simulink model "rct_pendulum_pluspos"  (R2023a)
settings: Solver=FixedStepAuto  StartTime=0.0  StopTime=30  FixedStep=0.00005  MaxStep=1e-5  RelTol=1e-5  EnableMultiTasking=on
model workspace (MATLAB code in the model file):
  | mCart = 1;
  | mPend = 1;
  | g = 9.81;
  | L = 0.5;
  | theta0 = 0;
  | Kd = 10;
undefined symbols (not defined in the file): X, Y, Z
libraries: sm_lib x11, nesl_utility x5
settings Model: Creator=The MathWorks, Inc.  LastModifiedBy=kimdi
settings SolverCC: AlgebraicLoopSolver=TrustRegion  MaxZcPerStep=1
settings DataIOCC: LimitDataPoints=on  SaveFormat=Array  ReturnWorkspaceOutputs=off  OutputOption=SpecifiedOutputTimes  OutputTimes=0:1/30:12
settings OptimizationCC: ReuseModelBlockBuffer=off  LifeSpan=inf
settings DebuggingCC: UnderspecifiedInitializationDetection=Classic  MergeDetectMultiDrivingBlocksExec=none  SolverPrmCheckMsg=warning  UnconnectedInputMsg=warning  UnconnectedOutputMsg=warning  UnconnectedLineMsg=warning  StateNameClashWarn=warning  SFUnexpectedBacktrackingDiag=warning  SFNoUnconditionalDefaultTransitionDiag=warning  SFExecutionAtInitializationDiag=none  ArithmeticOperatorsInVariantConditions=warning
settings HardwareCC: ProdBitPerPointer=32  ProdBitPerSizeT=32  ProdBitPerPtrDiffT=32  ProdLargestAtomicFloat=None  ProdIntDivRoundTo=Undefined  ProdEndianess=Unspecified  ProdWordSize=32  ProdHWDeviceType=32-bit Generic
settings ModelReferenceCC: EnableRefExpFcnMdlSchedulingChecks=on  PropagateSignalLabelsOutOfModel=off
settings SFSimCC: SimUseLocalCustomCode=off  CustomCodeUndefinedFunction=UseInterfaceOnly
settings RTWCC: RTWUseLocalCustomCode=off  DLArmComputeVersion=19.05
settings CodeAppCC: StateflowObjectComments=on
settings GRTTargetCC: TargetLangStandard=C89/C90 (ANSI)
settings ConfigComp: CovMetricSettings=dw  CovSaveCumulativeToWorkspaceVar=on  CovSaveSingleToWorkspaceVar=on  CovExternalEMLEnable=off  CovSFcnEnable=off
settings SimscapeCC: SimscapeNormalizeSystem=off
settings ConfigurationSet: Description=SimMechanics 2G
settings ExplorerConfigSet: InternalSimMechanicsExplorerSettings="<ExplorerConfiguration><canonicalview>default</canonicalview><TilePanel><TileInfo><Tiles Columns=\"1\" Count=\"1\" Rows=\"1\"><Column Left=\"2\" Weight=\"1\"/><Column Left=\"591\"/><Row Top=\"2\" Weight=\"1\"/><Row Top=\"389\"/><Tile Height=\"1\" Width=\"1\" X=\"0\" Y=\"0\"/></Tiles></TileInfo><SceneInfo><SceneViewer><BGColor><R>0.60000002384185791</R><G>0.60000002384185791</G><B>0.60000002384185791</B></BGColor><Camera><Position><X>0.64243946887929204</X><Y>-49.663614699976236</Y><Z>0.22319801622928798</Z></Position><Center><X>0.64243946887929204</X><Y>0</Y><Z>0.22319801622928798</Z></Center><Up><X>0</X><Y>-0</Y><Z>1</Z></Up><Left>-0.88124258449330872</Left><Right>0.88124258449330872</Right><Bottom>-0.30475961919215644</Bottom><Top>0.30475961919215644</Top></Camera></SceneViewer></SceneInfo></TilePanel></ExplorerConfiguration>"

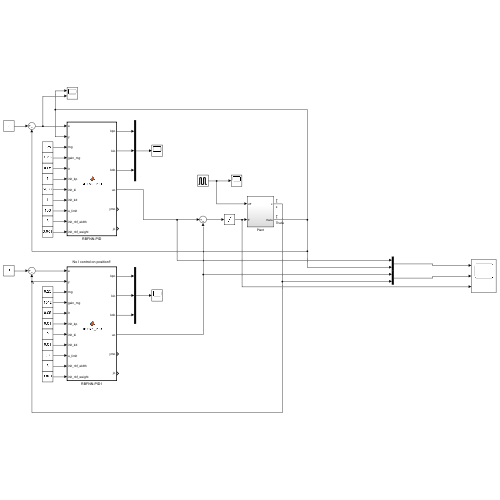
[thumbnail: Simulink's stored preview of the top-level diagram]
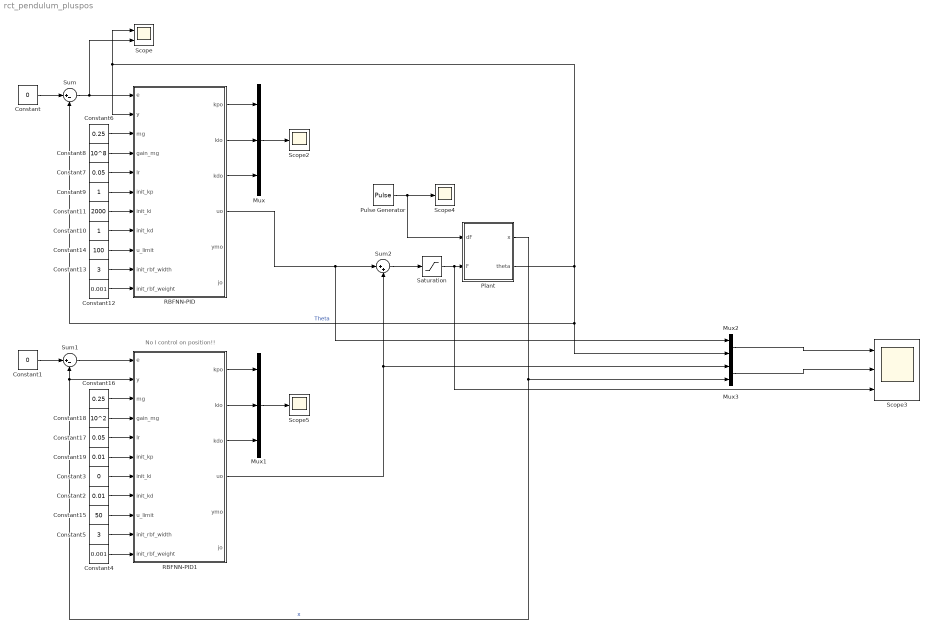
== system rct_pendulum_pluspos ==
  note: No I control on position!!
  Constant : Constant  Value=0
  Constant1 : Constant  Value=0
  Constant10 : Constant
  Constant11 : Constant  Value=2000
  Constant12 : Constant  Value=0.001
  Constant13 : Constant  Value=3
  Constant14 : Constant  Value=100
  Constant15 : Constant  Value=50
  Constant16 : Constant  Value=0.25
  Constant17 : Constant  Value=0.05
  Constant18 : Constant  Value=10^2
  Constant19 : Constant  Value=0.01
  Constant2 : Constant  Value=0.01
  Constant3 : Constant  Value=0
  Constant4 : Constant  Value=0.001
  Constant5 : Constant  Value=3
  Constant6 : Constant  Value=0.25
  Constant7 : Constant  Value=0.05
  Constant8 : Constant  Value=10^8
  Constant9 : Constant
  Mux : Mux  Inputs=3
  Mux1 : Mux  Inputs=3
  Mux2 : Mux  Inputs=2
  Mux3 : Mux  Inputs=2
  Plant : Subsystem
  Pulse Generator : DiscretePulseGenerator  PulseType=Time based  Period=10  PulseWidth=5  PhaseDelay=3
  RBFNN-PID : MATLAB Function  TreatAsAtomicUnit=on
  RBFNN-PID1 : MATLAB Function  TreatAsAtomicUnit=on
  Saturation : Saturate  UpperLimit=1000  LowerLimit=-1000
  Scope : Scope  NumInputPorts=2
  Scope2 : Scope
  Scope3 : Scope  NumInputPorts=3
  Scope4 : Scope
  Scope5 : Scope
  Sum : Sum  Inputs=|+-
  Sum1 : Sum  Inputs=|+-
  Sum2 : Sum  Inputs=|++
  wires:
  Constant/1 -> Sum/1
  Sum/1 -> RBFNN-PID/1(e), Scope/2
  Plant/2(theta) -> RBFNN-PID/2(y), Scope/1, Sum/2, Mux2/2  "Theta"
  Mux/1 -> Scope2/1
  RBFNN-PID/1(kpo) -> Mux/1
  RBFNN-PID/2(kio) -> Mux/2
  RBFNN-PID/3(kdo) -> Mux/3
  Constant1/1 -> Sum1/1
  Sum1/1 -> RBFNN-PID1/1(e)
  Plant/1(x) -> RBFNN-PID1/2(y), Sum1/2, Mux3/2  "x"
  RBFNN-PID1/3(kdo) -> Mux1/3
  Mux1/1 -> Scope5/1
  RBFNN-PID1/2(kio) -> Mux1/2
  RBFNN-PID1/1(kpo) -> Mux1/1
  RBFNN-PID/4(uo) -> Sum2/1, Mux2/1
  RBFNN-PID1/4(uo) -> Mux3/1, Sum2/2
  Mux2/1 -> Scope3/1
  Mux3/1 -> Scope3/2
  Pulse Generator/1 -> Plant/1(dF), Scope4/1
  Saturation/1 -> Scope3/3, Plant/2(F)
  Sum2/1 -> Saturation/1
  Constant6/1 -> RBFNN-PID/3(mg)
  Constant8/1 -> RBFNN-PID/4(gain_mg)
  Constant7/1 -> RBFNN-PID/5(lr)
  Constant9/1 -> RBFNN-PID/6(init_kp)
  Constant10/1 -> RBFNN-PID/8(init_kd)
  Constant11/1 -> RBFNN-PID/7(init_ki)
  Constant13/1 -> RBFNN-PID/10(init_rbf_width)
  Constant14/1 -> RBFNN-PID/9(u_limit)
  Constant12/1 -> RBFNN-PID/11(init_rbf_weight)
  Constant16/1 -> RBFNN-PID1/3(mg)
  Constant3/1 -> RBFNN-PID1/7(init_ki)
  Constant15/1 -> RBFNN-PID1/9(u_limit)
  Constant5/1 -> RBFNN-PID1/10(init_rbf_width)
  Constant4/1 -> RBFNN-PID1/11(init_rbf_weight)
  Constant17/1 -> RBFNN-PID1/5(lr)
  Constant19/1 -> RBFNN-PID1/6(init_kp)
  Constant2/1 -> RBFNN-PID1/8(init_kd)
  Constant18/1 -> RBFNN-PID1/4(gain_mg)

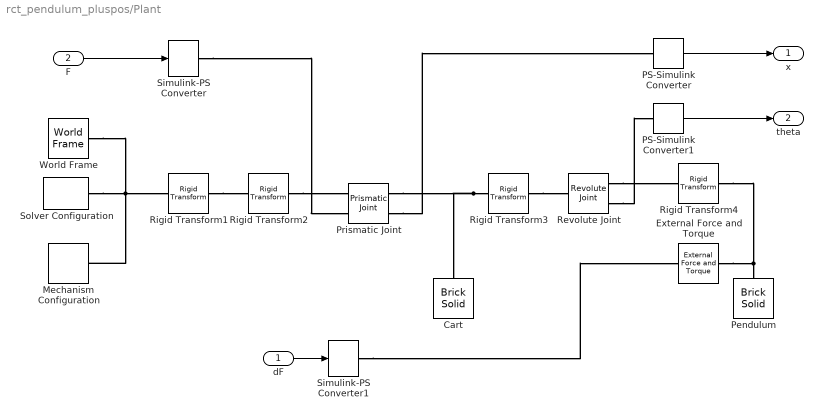
== system rct_pendulum_pluspos/Plant ==
  dF : Inport
  F : Inport  Port=2
  Cart : sm_lib/Body Elements/Brick Solid  GraphicAmbientColor=[0.15 0.15 0.15 1.0]  BasedOnType=Mass  BrickDimensions=[L/6 L/6 L/3]  BrickDimensionsUnits=m  CenterOfMass=[0 0 0]  CenterOfMassUnits=m  GraphicDiffuseColor=[0.5 0.5 0.5]  Density=1000  DensityUnits=kg/(m^3)  DoExposeReferenceFrame=on  GraphicEmissiveColor=[0.0 0.0 0.0 1.0]  ExportEntireGeometry=off  SerializedFrames=<Frames/>  MarkerShape=Sphere  MarkerSize=10  GraphicType=FromGeometry  InertiaType=PointMass  Mass=mCart  MassUnits=kg  MomentsOfInertia=[1 1 1]  MomentsOfInertiaUnits=kg*m^2  GraphicOpacity=1.0  ProductsOfInertia=[0 0 0]  ProductsOfInertiaUnits=kg*m^2  GraphicShininess=75  GraphicSpecularColor=[0.5 0.5 0.5 1.0]  GraphicVisPropType=SimpleVisualProperties
  External Force and Torque : sm_lib/Forces and Torques/External Force and Torque  ForceResolutionFrame=World  EnableForceX=on  EnableForceY=off  EnableForceZ=off  EnableForce=off  TorqueResolutionFrame=AttachedFrame  EnableTorqueX=off  EnableTorqueY=off  EnableTorqueZ=off  EnableTorque=off
  Mechanism Configuration : sm_lib/Utilities/Mechanism Configuration  UniformGravity=Constant  GravityVector=[0 0 -9.81]  GravityVectorUnits=m/s^2  LinearizationDelta=0.001  JointModeTransitionNonlinearIterations=2
  PS-Simulink Converter : nesl_utility/PS-Simulink Converter  PhysicalDomain=network_engine_domain  SubClassName=ps_output  LeftPortType=input  RightPortType=output  PseudoPeriodic=off  Frequencies=[]  VectorFormat=1-D array  Unit=1  AffineConversion=off
  PS-Simulink Converter1 : nesl_utility/PS-Simulink Converter  PhysicalDomain=network_engine_domain  SubClassName=ps_output  LeftPortType=input  RightPortType=output  PseudoPeriodic=off  Frequencies=[]  VectorFormat=1-D array  Unit=1  AffineConversion=off
  Pendulum : sm_lib/Body Elements/Brick Solid  GraphicAmbientColor=[0.15 0.15 0.15 1.0]  BasedOnType=Mass  BrickDimensions=[L L/12 L/12]  BrickDimensionsUnits=m  CenterOfMass=[0 0 0]  CenterOfMassUnits=m  GraphicDiffuseColor=[0.8 0.0 0.2]  Density=1000  DensityUnits=kg/(m^3)  DoExposeReferenceFrame=on  GraphicEmissiveColor=[0.0 0.0 0.0 1.0]  ExportEntireGeometry=off  SerializedFrames=<Frames/>  MarkerShape=Sphere  MarkerSize=10  GraphicType=FromGeometry  InertiaType=PointMass  Mass=mPend  MassUnits=kg  MomentsOfInertia=[1 1 1]  MomentsOfInertiaUnits=kg*m^2  GraphicOpacity=1.0  ProductsOfInertia=[0 0 0]  ProductsOfInertiaUnits=kg*m^2  GraphicShininess=75  GraphicSpecularColor=[0.5 0.5 0.5 1.0]  GraphicVisPropType=SimpleVisualProperties
  Prismatic Joint : sm_lib/Joints/Prismatic Joint  JointMode=Normal  SenseConstraintForce=off  SenseConstraintForceX=off  SenseConstraintForceY=off  SenseConstraintForceZ=off  SenseConstraintTorque=off  SenseConstraintTorqueX=off  SenseConstraintTorqueY=off  SenseConstraintTorqueZ=off  SenseTotalForce=off  SenseTotalForceX=off  SenseTotalForceY=off  SenseTotalForceZ=off  SenseTotalTorque=off  SenseTotalTorqueX=off  SenseTotalTorqueY=off  SenseTotalTorqueZ=off  CompositeWrenchDir=FollowerOnBase  CompositeWrenchFrame=BaseFrame  EquilibriumPosition=0  EquilibriumPositionUnits=m  SpringStiffness=0  SpringStiffnessUnits=N/m  DampingCoefficient=Kd  DampingCoefficientUnits=N/(m/s)  TorqueActuationMode=InputTorque  MotionActuationMode=ComputedMotion  SensePosition=on  SenseVelocity=off  SenseAcceleration=off  SenseTorqueForce=off  SenseLowerLimitTorqueForce=off  SenseUpperLimitTorqueForce=off  LowerLimitSpecify=off  LowerLimitBound=-1  LowerLimitBoundUnits=m  LowerLimitStiffness=1e6  LowerLimitStiffnessUnits=N/m  LowerLimitDamping=1e3  LowerLimitDampingUnits=N/(m/s)  LowerLimitTransitionRegionWidth=1e-4  LowerLimitTransitionRegionWidthUnits=m  UpperLimitSpecify=off  UpperLimitBound=1  UpperLimitBoundUnits=m  UpperLimitStiffness=1e6  UpperLimitStiffnessUnits=N/m  UpperLimitDamping=1e3  UpperLimitDampingUnits=N/(m/s)  UpperLimitTransitionRegionWidth=1e-4  UpperLimitTransitionRegionWidthUnits=m  PositionTargetSpecify=off  PositionTargetPriority=High  PositionTargetValue=0  PositionTargetValueUnits=m  VelocityTargetSpecify=off  VelocityTargetPriority=High  VelocityTargetValue=0  VelocityTargetValueUnits=m/s
  Revolute Joint : sm_lib/Joints/Revolute Joint  JointMode=Normal  SenseConstraintForce=off  SenseConstraintForceX=off  SenseConstraintForceY=off  SenseConstraintForceZ=off  SenseConstraintTorque=off  SenseConstraintTorqueX=off  SenseConstraintTorqueY=off  SenseConstraintTorqueZ=off  SenseTotalForce=off  SenseTotalForceX=off  SenseTotalForceY=off  SenseTotalForceZ=off  SenseTotalTorque=off  SenseTotalTorqueX=off  SenseTotalTorqueY=off  SenseTotalTorqueZ=off  CompositeWrenchDir=FollowerOnBase  CompositeWrenchFrame=BaseFrame  EquilibriumPosition=0  EquilibriumPositionUnits=deg  SpringStiffness=0  SpringStiffnessUnits=N*m/deg  DampingCoefficient=0  DampingCoefficientUnits=N*m/(rad/s)  TorqueActuationMode=NoTorque  MotionActuationMode=ComputedMotion  SensePosition=on  SenseVelocity=off  SenseAcceleration=off  SenseTorqueForce=off  SenseLowerLimitTorqueForce=off  SenseUpperLimitTorqueForce=off  LowerLimitSpecify=off  LowerLimitBound=-90  LowerLimitBoundUnits=deg  LowerLimitStiffness=1e4  LowerLimitStiffnessUnits=N*m/deg  LowerLimitDamping=10  LowerLimitDampingUnits=N*m/(deg/s)  LowerLimitTransitionRegionWidth=0.1  LowerLimitTransitionRegionWidthUnits=deg  UpperLimitSpecify=off  UpperLimitBound=90  UpperLimitBoundUnits=deg  UpperLimitStiffness=1e4  UpperLimitStiffnessUnits=N*m/deg  UpperLimitDamping=10  UpperLimitDampingUnits=N*m/(deg/s)  UpperLimitTransitionRegionWidth=0.1  UpperLimitTransitionRegionWidthUnits=deg  PositionTargetSpecify=on  PositionTargetPriority=High  PositionTargetValue=theta0  PositionTargetValueUnits=deg  VelocityTargetSpecify=off  VelocityTargetPriority=High  VelocityTargetValue=0  VelocityTargetValueUnits=deg/s
  Rigid Transform1 : sm_lib/Frames and Transforms/Rigid Transform  TranslationMethod=None  TranslationStandardOffset=0  TranslationStandardOffsetUnits=m  TranslationStandardAxis=+Z  TranslationCartesianOffset=[0 0 0]  TranslationCartesianOffsetUnits=m  TranslationROffset=0  TranslationROffsetUnits=m  TranslationZOffset=0  TranslationZOffsetUnits=m  TranslationThetaOffset=0  TranslationThetaOffsetUnits=deg  RotationMethod=StandardAxis  RotationAngleUnits=deg  RotationStandardAxis=+Y  RotationAngle=90  RotationArbitraryAxis=[0 0 1]  FollAlignAxisA=+X  BaseAlignAxisA=+Y  FollAlignAxisB=+Y  BaseAlignAxisB=+Z  RotationSequenceAxes=FollowerAxes  RotationSequence=XYX  RotationSequenceAngles=[0 0 0]  RotationSequenceAnglesUnits=deg  RotationMatrix=[1 0 0; 0 1 0; 0 0 1]  Quaternion=[1 0 0 0]
  Rigid Transform2 : sm_lib/Frames and Transforms/Rigid Transform  TranslationMethod=None  TranslationStandardOffset=0  TranslationStandardOffsetUnits=m  TranslationStandardAxis=+Z  TranslationCartesianOffset=[0 0 0]  TranslationCartesianOffsetUnits=m  TranslationROffset=0  TranslationROffsetUnits=m  TranslationZOffset=0  TranslationZOffsetUnits=m  TranslationThetaOffset=0  TranslationThetaOffsetUnits=deg  RotationMethod=StandardAxis  RotationAngleUnits=deg  RotationStandardAxis=+Z  RotationAngle=180  RotationArbitraryAxis=[0 0 1]  FollAlignAxisA=+X  BaseAlignAxisA=+Y  FollAlignAxisB=+Y  BaseAlignAxisB=+Z  RotationSequenceAxes=FollowerAxes  RotationSequence=XYX  RotationSequenceAngles=[0 0 0]  RotationSequenceAnglesUnits=deg  RotationMatrix=[1 0 0; 0 1 0; 0 0 1]  Quaternion=[1 0 0 0]
  Rigid Transform3 : sm_lib/Frames and Transforms/Rigid Transform  TranslationMethod=None  TranslationStandardOffset=0  TranslationStandardOffsetUnits=m  TranslationStandardAxis=+Z  TranslationCartesianOffset=[0 0 0]  TranslationCartesianOffsetUnits=m  TranslationROffset=0  TranslationROffsetUnits=m  TranslationZOffset=0  TranslationZOffsetUnits=m  TranslationThetaOffset=0  TranslationThetaOffsetUnits=deg  RotationMethod=StandardAxis  RotationAngleUnits=deg  RotationStandardAxis=-X  RotationAngle=90  RotationArbitraryAxis=[0 0 1]  FollAlignAxisA=+X  BaseAlignAxisA=+Y  FollAlignAxisB=+Y  BaseAlignAxisB=+Z  RotationSequenceAxes=FollowerAxes  RotationSequence=XYX  RotationSequenceAngles=[0 0 0]  RotationSequenceAnglesUnits=deg  RotationMatrix=[1 0 0; 0 1 0; 0 0 1]  Quaternion=[1 0 0 0]
  Rigid Transform4 : sm_lib/Frames and Transforms/Rigid Transform  TranslationMethod=StandardAxis  TranslationStandardOffset=L/2  TranslationStandardOffsetUnits=m  TranslationStandardAxis=+X  TranslationCartesianOffset=[0 0 0]  TranslationCartesianOffsetUnits=m  TranslationROffset=0  TranslationROffsetUnits=m  TranslationZOffset=0  TranslationZOffsetUnits=m  TranslationThetaOffset=0  TranslationThetaOffsetUnits=deg  RotationMethod=StandardAxis  RotationAngleUnits=deg  RotationStandardAxis=+X  RotationAngle=90  RotationArbitraryAxis=[0 0 1]  FollAlignAxisA=+X  BaseAlignAxisA=+Y  FollAlignAxisB=+Y  BaseAlignAxisB=+Z  RotationSequenceAxes=FollowerAxes  RotationSequence=XYX  RotationSequenceAngles=[0 0 0]  RotationSequenceAnglesUnits=deg  RotationMatrix=[1 0 0; 0 1 0; 0 0 1]  Quaternion=[1 0 0 0]
  Simulink-PS Converter : nesl_utility/Simulink-PS Converter  PhysicalDomain=network_engine_domain  SubClassName=ps_input  LeftPortType=input  RightPortType=output  PseudoPeriodic=off  Frequencies=[]  NoiseDistribution=none  NoiseParameters=[]  Unit=1  AffineConversion=off  FilteringAndDerivatives=zero  SimscapeFilterOrder=1  InputFilterTimeConstant=0.001  UdotUserProvided=1
  Simulink-PS Converter1 : nesl_utility/Simulink-PS Converter  PhysicalDomain=network_engine_domain  SubClassName=ps_input  LeftPortType=input  RightPortType=output  PseudoPeriodic=off  Frequencies=[]  NoiseDistribution=none  NoiseParameters=[]  Unit=1  AffineConversion=off  FilteringAndDerivatives=zero  SimscapeFilterOrder=1  InputFilterTimeConstant=0.001  UdotUserProvided=1
  Solver Configuration : nesl_utility/Solver Configuration  PhysicalDomain=network_engine_domain  SubClassName=solver  LeftPortType=input  RightPortType=generic  Tones=[]  Harmonics=[]  SimulateNoise=off  Profile=off  UseLocalSampling=off  EnableSwitchedLinearOptims=on  FrequencyDomain=off  UseCCode=off  RelTol=0.001  AbsTol=1e-06  MinStep=1e-09  ToWorkspace=off  RevertToSquareIcSolve=off  NumHomotopyIterations=100  PhasorMode=off  PhasorModeNumHarmonics=1  ConsistencySolver=NEWTON_FTOL  IndexReductionMethod=DerivativeReplacement  DoDC=off  ResidualTolerance=1e-09  ConsistencyTolSource=GLOBAL  ConsistencyAbsTol=0.001  ConsistencyRelTol=0.001  ConsistencyTolFactor=0.001  UseLocalSolver=off  LocalSolverChoice=NE_BACKWARD_EULER_ADVANCER  ResolveIndetEquations=on  FunctionEvalNumThread=1  LocalSolverSampleTime=0.001  DoFixedCost=off  MaxNonlinIter=3  MaxModeIter=2  ComputeImpulses=off  ImpulseIterations=2  LinearAlgebra=Sparse  LinearAlgebraNumThread=0  EquationFormulation=NE_TIME_EF  DelaysMemoryBudget=1024  AutomaticFiltering=on  FilteringTimeConstant=0.001  PartitionStorageMethod=AS_NEEDED  PartitionMemoryBudget=1024  PartitionMethod=FAST
  World Frame : sm_lib/Frames and Transforms/World Frame
  x : Outport  VectorParamsAs1DForOutWhenUnconnected=off
  theta : Outport  Port=2  VectorParamsAs1DForOutWhenUnconnected=off
  wires:
  PS-Simulink Converter1/1 -> theta/1
  PS-Simulink Converter/1 -> x/1
  F/1 -> Simulink-PS Converter/1
  dF/1 -> Simulink-PS Converter1/1
  connections:
  Rigid Transform3/LConn1 -- Cart/RConn1 -- Prismatic Joint/RConn1
  World Frame/RConn1 -- Solver Configuration/RConn1 -- Mechanism Configuration/RConn1 -- Rigid Transform1/LConn1
  Revolute Joint/RConn1 -- Rigid Transform4/LConn1
  Rigid Transform4/RConn1 -- External Force and Torque/RConn1 -- Pendulum/RConn1
  Rigid Transform3/RConn1 -- Revolute Joint/LConn1
  Revolute Joint/RConn2 -- PS-Simulink Converter1/LConn1
  Prismatic Joint/RConn2 -- PS-Simulink Converter/LConn1
  Simulink-PS Converter/RConn1 -- Prismatic Joint/LConn2
  Simulink-PS Converter1/RConn1 -- External Force and Torque/LConn1
  Rigid Transform1/RConn1 -- Rigid Transform2/LConn1
  Rigid Transform2/RConn1 -- Prismatic Joint/LConn1

== matlab function rct_pendulum_pluspos/RBFNN-PID1 ==
  settings: updateMethod=DISCRETE
  data: e input; y input; kpo output; kio output; kdo output; mg input; gain_mg input; lr input; uo output; ymo output; jo output; init_kp input; init_ki input; init_kd input; u_limit input; init_rbf_width input; init_rbf_weight input
% e is error, PID input
% y is output of plant
% mg is momentum factor of RBF NN
% lr is learning rate of RBF NN
function [kpo, kio, kdo, uo, ymo, jo]= RBFNN_PID(e, y, mg, gain_mg, lr, init_kp, init_ki, init_kd, u_limit, init_rbf_width, init_rbf_weight)
persistent flag;

% PID controller parameters
persistent ek ek1 ek2; % e(k), e(k-1), e(k-2)
persistent sumek;
persistent xc1 xc2 xc3; % xc(1), xc(2), xc(3)
persistent u du;
persistent kp ki kd;

% RBF NN parameters
n = 3; % size of input
m = 8; % size of hidden
persistent X; % input X [n x 1]
persistent Ck Ck1 Ck2; % center vector C [m x n]
persistent H; % radial vector [m x 1]
persistent Bk Bk1 Bk2; % radial width vector B [m x 1]
persistent Wk Wk1 Wk2; % weight vector W [m x 1]
persistent yk yk1; % output of plant
persistent ym; % output of RBF NN
persistent J; % jacobian information of RBF NN

% initialize inital value just first time
if isempty(flag)
    flag = 1;

    ek1 = 0;
    ek2 = 0;
    sumek = 0;
    
    u = 0;
    du = 0;

    kp = init_kp;
    ki = init_ki;
    kd = init_kd;
    X = zeros(n, 1);
    Ck = zeros(m, n);
    Ck1 = zeros(m, n);
    Ck2 = zeros(m, n);
    H = zeros(m, 1);
    Bk = init_rbf_width * ones(m, 1) + rand(m, 1); %ones(m, 1);
    Bk1 = Bk;
    Bk2 = Bk;
    Wk = init_rbf_weight * ones(m, 1);
    Wk1 = Wk;
    Wk2 = Wk;

    yk1 = 0;
end

% set input vector
yk = y;
X(1) = u;
X(2) = yk;
X(3) = yk1;

% calculate centor vector
for j = 1:m
    dist = norm(X - Ck(j));
    H(j) = exp(-((dist^2) / (2 * Bk(j)^2)));
end

% calculate RBF NN parameters
ym = Wk' * H;
for j = 1:m
    dWk = mg * (yk - ym) * H(j);
    Wk(j) = Wk1(j) + dWk + lr * (Wk1(j) - Wk2(j));
    dBk = mg * (yk - ym) * Wk(j) * H(j) * ((norm(X - Ck(j))^2) / (Bk(j) ^ 3));
    Bk(j) = Bk1(j) + dBk + lr * (Bk1(j) - Bk2(j));
    for i = 1:n
        dCk = mg * (yk - ym) * Wk(j) * ((X(i) - Ck(j, i)) / (Bk(j)^2));
        Ck(j, i) = Ck1(j, i) + dCk + lr * (Ck1(j, i) - Ck2(j, i));
    end
end

% calculate RBF NN J
J = 0;
for j = 1:m
    J = J + Wk(j) * H(j) * ((Ck(j, 1) - X(1)) / Bk(j) ^ 2);
end
jo = J;


% ek is current error.
ek = e;
sumek = sumek + ek;

% calculate controller input
xc1 = ek - ek1;
xc2 = ek;
xc3 = ek - 2 * ek1 + ek2;

% update PID gain
kp = kp + gain_mg * mg * ek * J * xc1;
%ki = ki + gain_mg * mg * ek * J * xc2;
kd = kd + gain_mg * ek * J * xc3;

% calculate pid output
du = kp * xc1 + ki * xc2 + kd * xc3;
u = u + du;
if abs(u) > u_limit
    u = du;
end

uo = u;

% return output
kpo = kp;
kio = ki;
kdo = kd;
ymo = ym;

% in final, proceed time k, shift
ek1 = ek;
ek2 = ek1;
yk1 = yk;
Ck1 = Ck;
Ck2 = Ck1;
Bk1 = Bk;
Bk2 = Bk1;
Wk1 = Wk;
Wk2 = Wk1;

== matlab function rct_pendulum_pluspos/RBFNN-PID ==
  settings: updateMethod=DISCRETE
  data: e input; y input; kpo output; kio output; kdo output; mg input; gain_mg input; lr input; uo output; ymo output; jo output; init_kp input; init_ki input; init_kd input; u_limit input; init_rbf_width input; init_rbf_weight input
% e is error, PID input
% y is output of plant
% mg is momentum factor of RBF NN
% lr is learning rate of RBF NN
function [kpo, kio, kdo, uo, ymo, jo]= RBFNN_PID(e, y, mg, gain_mg, lr, init_kp, init_ki, init_kd, u_limit, init_rbf_width, init_rbf_weight)
persistent flag;

% PID controller parameters
persistent ek ek1 ek2; % e(k), e(k-1), e(k-2)
persistent sumek;
persistent xc1 xc2 xc3; % xc(1), xc(2), xc(3)
persistent u du;
persistent kp ki kd;

% RBF NN parameters
n = 3; % size of input
m = 8; % size of hidden
persistent X; % input X [n x 1]
persistent Ck Ck1 Ck2; % center vector C [m x n]
persistent H; % radial vector [m x 1]
persistent Bk Bk1 Bk2; % radial width vector B [m x 1]
persistent Wk Wk1 Wk2; % weight vector W [m x 1]
persistent yk yk1; % output of plant
persistent ym; % output of RBF NN
persistent J; % jacobian information of RBF NN

% initialize inital value just first time
if isempty(flag)
    flag = 1;

    ek1 = 0;
    ek2 = 0;
    sumek = 0;
    
    u = 0;
    du = 0;

    kp = init_kp;
    ki = init_ki;
    kd = init_kd;
    X = zeros(n, 1);
    Ck = zeros(m, n);
    Ck1 = zeros(m, n);
    Ck2 = zeros(m, n);
    H = zeros(m, 1);
    Bk = init_rbf_width * ones(m, 1) + rand(m, 1); %ones(m, 1);
    Bk1 = Bk;
    Bk2 = Bk;
    Wk = init_rbf_weight * ones(m, 1);
    Wk1 = Wk;
    Wk2 = Wk;

    yk1 = 0;
end

% set input vector
yk = y;
X(1) = u;
X(2) = yk;
X(3) = yk1;

% calculate centor vector
for j = 1:m
    dist = norm(X - Ck(j));
    H(j) = exp(-((dist^2) / (2 * Bk(j)^2)));
end

% calculate RBF NN parameters
ym = Wk' * H;
for j = 1:m
    dWk = mg * (yk - ym) * H(j);
    Wk(j) = Wk1(j) + dWk + lr * (Wk1(j) - Wk2(j));
    dBk = mg * (yk - ym) * Wk(j) * H(j) * ((norm(X - Ck(j))^2) / (Bk(j) ^ 3));
    Bk(j) = Bk1(j) + dBk + lr * (Bk1(j) - Bk2(j));
    for i = 1:n
        dCk = mg * (yk - ym) * Wk(j) * ((X(i) - Ck(j, i)) / (Bk(j)^2));
        Ck(j, i) = Ck1(j, i) + dCk + lr * (Ck1(j, i) - Ck2(j, i));
    end
end

% calculate RBF NN J
J = 0;
for j = 1:m
    J = J + Wk(j) * H(j) * ((Ck(j, 1) - X(1)) / Bk(j) ^ 2);
end
jo = J;


% ek is current error.
ek = e;
sumek = sumek + ek;

% calculate controller input
xc1 = ek - ek1;
xc2 = ek;
xc3 = ek - 2 * ek1 + ek2;

% update PID gain
kp = kp + gain_mg * mg * ek * J * xc1;
ki = ki + gain_mg * mg * ek * J * xc2;
kd = kd + gain_mg * ek * J * xc3;

% calculate pid output
du = kp * xc1 + ki * xc2 + kd * xc3;
u = u + du;
if abs(u) > u_limit
    u = du;
end

uo = u;

% return output
kpo = kp;
kio = ki;
kdo = kd;
ymo = ym;

% in final, proceed time k, shift
ek1 = ek;
ek2 = ek1;
yk1 = yk;
Ck1 = Ck;
Ck2 = Ck1;
Bk1 = Bk;
Bk2 = Bk1;
Wk1 = Wk;
Wk2 = Wk1;
